simulink model "model"  (R2019b)
settings: Solver=VariableStepAuto  StartTime=0.0  StopTime=800  RelTol=1e-3
values from neighbouring files (symbols this model uses):
  xi = [v_ini, gamma_ini, h_ini, phi_ini, theta_ini, q_ini, consumed_prop_ini, params.retro_rockets.max_thrust]    [run.m]
undefined symbols (not defined in the file or in its folder): Atm, Mars, params, Vehicle
settings Model: Creator=louis  LastModifiedBy=CHANDON
settings DebuggingCC: ArithmeticOperatorsInVariantConditions=warning
settings SFSimCC: CustomCodeUndefinedFunction=UseInterfaceOnly

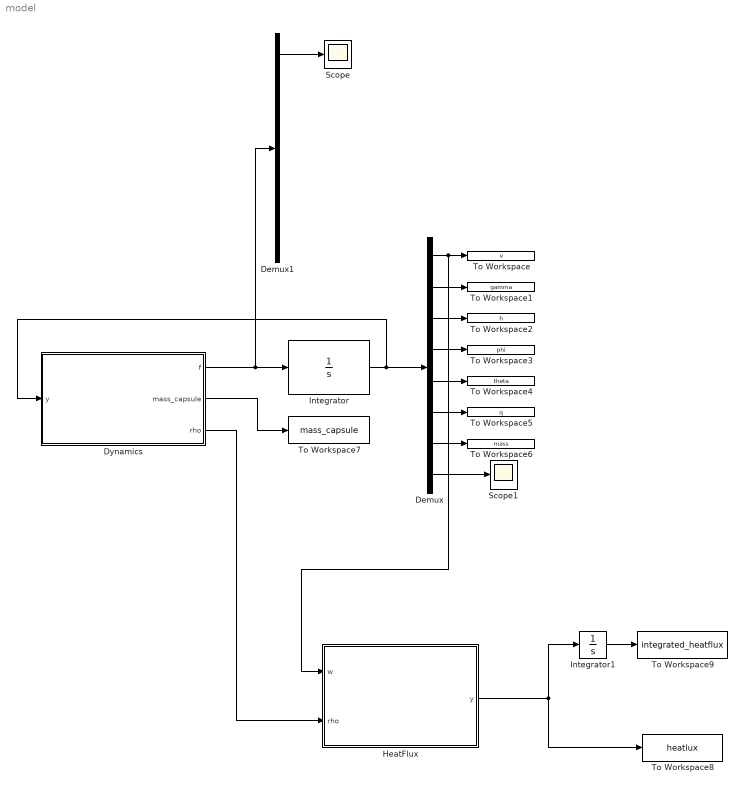
== system model ==
  Demux : Demux  Outputs=8
  Demux1 : Demux  Outputs=7
  Dynamics : MATLAB Function  TreatAsAtomicUnit=on
  HeatFlux : MATLAB Function  TreatAsAtomicUnit=on
  Integrator : Integrator  InitialCondition=xi
  Integrator1 : Integrator
  Scope : Scope
  Scope1 : Scope
  To Workspace : ToWorkspace  VariableName=v  SaveFormat=Timeseries  SampleTime=-1
  To Workspace1 : ToWorkspace  VariableName=gamma  SaveFormat=Timeseries  SampleTime=-1
  To Workspace2 : ToWorkspace  VariableName=h  SaveFormat=Timeseries  SampleTime=-1
  To Workspace3 : ToWorkspace  VariableName=phi  SaveFormat=Timeseries  SampleTime=-1
  To Workspace4 : ToWorkspace  VariableName=theta  SaveFormat=Timeseries  SampleTime=-1
  To Workspace5 : ToWorkspace  VariableName=q  SaveFormat=Timeseries  SampleTime=-1
  To Workspace6 : ToWorkspace  VariableName=mass  SaveFormat=Timeseries  SampleTime=-1
  To Workspace7 : ToWorkspace  VariableName=mass_capsule  SaveFormat=Timeseries  SampleTime=-1
  To Workspace8 : ToWorkspace  VariableName=heatlux  SaveFormat=Timeseries  SampleTime=-1
  To Workspace9 : ToWorkspace  VariableName=integrated_heatflux  SaveFormat=Timeseries  SampleTime=-1
  wires:
  Dynamics/1(f) -> Demux1/1, Integrator/1
  Integrator/1 -> Dynamics/1(y), Demux/1
  Demux/1 -> HeatFlux/1(w), To Workspace/1
  Demux/2 -> To Workspace1/1
  Demux/3 -> To Workspace2/1
  Demux/4 -> To Workspace3/1
  Demux/5 -> To Workspace4/1
  Demux/6 -> To Workspace5/1
  Demux1/1 -> Scope/1
  Demux/7 -> To Workspace6/1
  Dynamics/2(mass_capsule) -> To Workspace7/1
  Demux/8 -> Scope1/1
  Dynamics/3(rho) -> HeatFlux/2(rho)
  HeatFlux/1(y) -> To Workspace8/1, Integrator1/1
  Integrator1/1 -> To Workspace9/1

== matlab function model/HeatFlux ==
  data: y output; w input; Atm parameter; Vehicle parameter; rho input
function y = HeatFlux(w, Atm, Vehicle, rho)
    B_c = 9823.4;
    X_c = 3.158;
    Psi_c = 0.5;
    B_r = 1135.7;
    X_r = 8.5;
    Psi_r = 1.6;
    rho_SL = Atm.rho0;
    w = w * 1e-3;
    dq_conv = B_c * (w/3.048)^X_c * (rho/rho_SL)^Psi_c * sqrt(0.3048/Vehicle.r_n);
    dq_rad = B_r * (w/3.048)^X_r * (rho/rho_SL)^Psi_r * Vehicle.r_n/0.3048;
    
y = dq_conv + dq_rad;

== matlab function model/Dynamics ==
  data: y input; f output; Mars parameter; Atm parameter; Vehicle parameter; params parameter; mass_capsule output; rho output
function [f, mass_capsule, rho] = Dynamics(y, Mars, Atm, Vehicle, params)
    % Assignations
    v = y(1);
    gamma = y(2);
    h = y(3);
    phi = y(4);
    theta = y(5);
    q = y(6);
    if (y(7) < Vehicle.propellant)
        consumed_propellant = y(7);
    else
        consumed_propellant = Vehicle.propellant;
    end
    throttle = y(8);
    f = [0; 0; 0; 0; 0; 0; 0; 0];
    
    % Intermediate calculation
    thrust = 0;
    r = h + Mars.radius;
    g = Mars.mu / r.^2; % m/s^2 - Gravitationnal acceleration at r
    rho =  Atm.rho0 * exp(-h/Atm.hs);
    Pdyn = (1/2) .* rho .* v.^2; % Dynamic p ressure
    alpha = theta - gamma;
    if (h > params.parachute.at)
        mass_capsule = Vehicle.mass - consumed_propellant;
    elseif(h <= params.parachute.at > params.retro_rockets.at)
        mass_capsule = Vehicle.mass - consumed_propellant - Vehicle.Heatshield.mass;
    else
        mass_capsule = Vehicle.mass - consumed_propellant - Vehicle.Heatshield.mass - Vehicle.Parachute.mass;
    end
    
    if (params.controlled && h > params.parachute.at)
        B = (Vehicle.S .* Vehicle.CD) ./ (mass_capsule);
        dv_aero = params.v_des - sqrt(v.^2+((2.*Mars.mu).*((1./params.r_des)-(1./r))));
        gamma_ref = asin((1/2).*B.*Atm.hs.*((params.rho_des - rho) ./ log(1 + dv_aero./v)));
        
        k = (Pdyn .* Vehicle.S .* Vehicle.CL) ./ (v .* mass_capsule);
        theta_eq = gamma - (cos(gamma) .* mass_capsule) ./ (Pdyn.*Vehicle.S.*Vehicle.CL) .* (v.^2 ./ r - Mars.mu./r.^2);
        theta_cmd = theta_eq + (1./(params.tau.*k)) .* (gamma_ref - gamma);
        
        % saturation
        if (theta_cmd > deg2rad(60))
            theta_cmd = deg2rad(60);
        end
        
        Kp = params.wn.^2;
        Kd = 2 * params.zeta .* params.wn;
        k = (Vehicle.CMdelta .* Pdyn * Vehicle.S * Vehicle.d) / Vehicle.J;
        delta_eq = (-Vehicle.CMalpha/Vehicle.CMdelta) .* (theta - gamma) - (Vehicle.CMq .* Vehicle.d .* q) ./ (2 .* v .* Vehicle.CMdelta);
        delta_cmd = delta_eq + Kp./k .* (theta_cmd - theta) + Kd./k .* (-q);
    else
        delta_cmd = 0;
    end
    
    Daero = Pdyn .* Vehicle.S .* Vehicle.CD;
    Laero = Pdyn .* Vehicle.S .* Vehicle.CL .* alpha;
    Maero = Pdyn .* Vehicle.S .* Vehicle.d .* (Vehicle.CMalpha .* alpha + (Vehicle.d / (2.*v)) .* Vehicle.CMq.*q + Vehicle.CMdelta.*delta_cmd); 
    
    if (h <= params.parachute.at && h >= params.retro_rockets.at)
        Daero = Daero + Vehicle.Parachute.CD .* ((rho .* v.^2) / 2) * Vehicle.Parachute.S;
        Laero = 0;
    end
    
    if (h <= 0)
        f(1) = 0;
    elseif (h <= params.parachute.at && h >= params.retro_rockets.at)
        f(1) = (-Daero) / mass_capsule + g;
    elseif (h <= params.retro_rockets.at && consumed_propellant < Vehicle.propellant && h > 0 && v > 1)
        thrust = throttle;
        if (thrust > params.retro_rockets.max_thrust)
            thrust = params.retro_rockets.max_thrust;
        end
        if (v <= 1)
            thrust = -mass_capsule * g;
        end
        f(1) = -thrust / mass_capsule + g;
    else
        f(1) = (-Daero) / mass_capsule - g*sin(gamma);
    end
    
    f(2) = (1/v) * (Laero/mass_capsule + ((v.^2/r) - g)*cos(gamma));

    if (h <= 0)
        f(3) = 0;
    elseif (h <= params.parachute.at)
        f(3) = -v;
    else
        f(3) = v * sin(gamma);
    end
    
    if (h <= 0)
        f(4) = 0;
    else
        f(4) = v/r * cos(gamma);
    end
    f(5) = q;
    f(6) = (1 / Vehicle.J) * Maero;
    if (h <= params.retro_rockets.at && h > 0 && consumed_propellant < Vehicle.propellant)
        flow_rate = thrust / params.retro_rockets.exhaust_velocity;
        f(7) = flow_rate;
        f(8) = -mass_capsule*(1/y(8))-g;
    end
    f = f(:);
end
